simulink model "baseline_carlaClosedLoopPipeline"  (R2026a)
settings: Solver=FixedStepAuto  StopTime=300  FixedStep=0.1
settings Model: Creator=ADITYA  LastModifiedBy=ADITYA

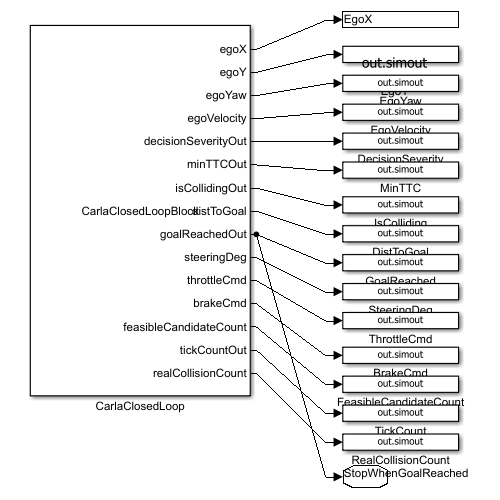
[thumbnail: Simulink's stored preview of the top-level diagram]
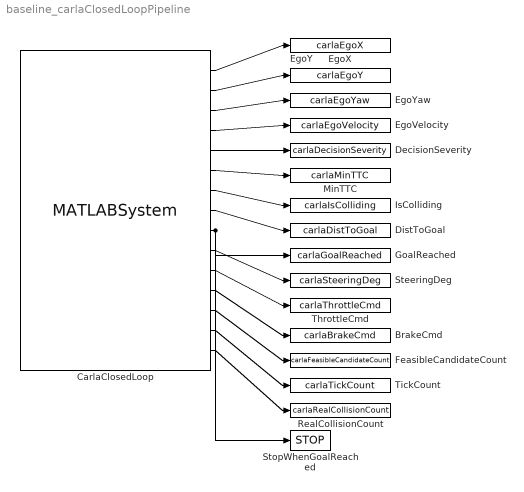
== system baseline_carlaClosedLoopPipeline ==
  BrakeCmd : ToWorkspace  VariableName=carlaBrakeCmd  SampleTime=-1
  CarlaClosedLoop : MATLABSystem  System=CarlaClosedLoopBlock  TurnRadiusM=12.0  ApproachLengthM=45.0  ExitLengthM=25.0  ExitHeadingDeg=89.64  BaseSpeedMps=4.0  SensorRangeM=25.0  GoalToleranceM=3.0  SimulateUsing=Interpreted execution
      mask Type: CarlaClosedLoopBlock
  DecisionSeverity : ToWorkspace  VariableName=carlaDecisionSeverity  SampleTime=-1
  DistToGoal : ToWorkspace  VariableName=carlaDistToGoal  SampleTime=-1
  EgoVelocity : ToWorkspace  VariableName=carlaEgoVelocity  SampleTime=-1
  EgoX : ToWorkspace  VariableName=carlaEgoX  SampleTime=-1
  EgoY : ToWorkspace  VariableName=carlaEgoY  SampleTime=-1
  EgoYaw : ToWorkspace  VariableName=carlaEgoYaw  SampleTime=-1
  FeasibleCandidateCount : ToWorkspace  VariableName=carlaFeasibleCandidateCount  SampleTime=-1
  GoalReached : ToWorkspace  VariableName=carlaGoalReached  SampleTime=-1
  IsColliding : ToWorkspace  VariableName=carlaIsColliding  SampleTime=-1
  MinTTC : ToWorkspace  VariableName=carlaMinTTC  SampleTime=-1
  RealCollisionCount : ToWorkspace  VariableName=carlaRealCollisionCount  SampleTime=-1
  SteeringDeg : ToWorkspace  VariableName=carlaSteeringDeg  SampleTime=-1
  StopWhenGoalReached : Stop
  ThrottleCmd : ToWorkspace  VariableName=carlaThrottleCmd  SampleTime=-1
  TickCount : ToWorkspace  VariableName=carlaTickCount  SampleTime=-1
  wires:
  CarlaClosedLoop/1 -> EgoX/1
  CarlaClosedLoop/2 -> EgoY/1
  CarlaClosedLoop/3 -> EgoYaw/1
  CarlaClosedLoop/4 -> EgoVelocity/1
  CarlaClosedLoop/5 -> DecisionSeverity/1
  CarlaClosedLoop/6 -> MinTTC/1
  CarlaClosedLoop/7 -> IsColliding/1
  CarlaClosedLoop/8 -> DistToGoal/1
  CarlaClosedLoop/9 -> GoalReached/1, StopWhenGoalReached/1
  CarlaClosedLoop/10 -> SteeringDeg/1
  CarlaClosedLoop/11 -> ThrottleCmd/1
  CarlaClosedLoop/12 -> BrakeCmd/1
  CarlaClosedLoop/13 -> FeasibleCandidateCount/1
  CarlaClosedLoop/14 -> TickCount/1
  CarlaClosedLoop/15 -> RealCollisionCount/1
